simulink model "p3_rakete"  (R2015a)
settings: Solver=ode45  StartTime=0.0  StopTime=10.0  RelTol=1e-3
settings Model: Creator=leon  LastModifiedBy=leon

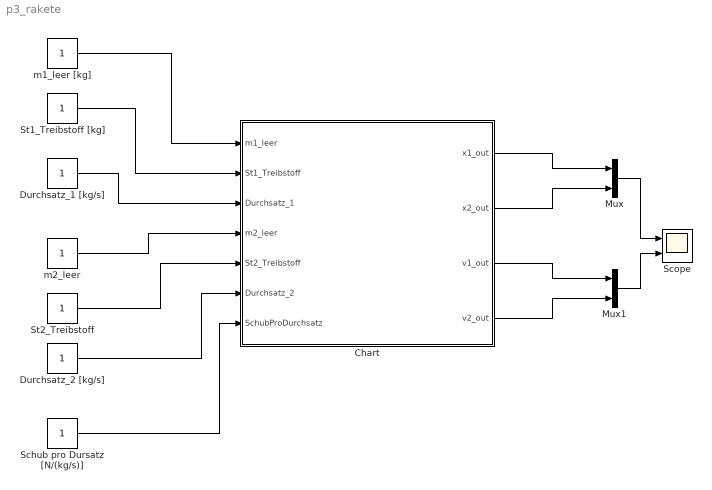
== system p3_rakete ==
  Chart : Stateflow chart  TreatAsAtomicUnit=on
  Durchsatz_1 [kg/s] : Constant
  Durchsatz_2 [kg/s] : Constant
  Mux : Mux  Inputs=2
  Mux1 : Mux  Inputs=2
  "Schub pro Dursatz [N/(kg/s)] " : Constant
  Scope : Scope  NumInputPorts=2
      settings: YMin=-5~-5  YMax=5~5
  St1_Treibstoff [kg] : Constant
  St2_Treibstoff : Constant
  "m1_leer [kg] " : Constant
  m2_leer : Constant
  wires:
  "m1_leer [kg] "/1 -> Chart/1(m1_leer)
  St1_Treibstoff [kg]/1 -> Chart/2(St1_Treibstoff)
  Durchsatz_1 [kg/s]/1 -> Chart/3(Durchsatz_1)
  m2_leer/1 -> Chart/4(m2_leer)
  St2_Treibstoff/1 -> Chart/5(St2_Treibstoff)
  Durchsatz_2 [kg/s]/1 -> Chart/6(Durchsatz_2)
  "Schub pro Dursatz [N/(kg/s)] "/1 -> Chart/7(SchubProDurchsatz)
  Chart/1(x1_out) -> Mux/1
  Chart/2(x2_out) -> Mux/2
  Chart/3(v1_out) -> Mux1/1
  Chart/4(v2_out) -> Mux1/2
  Mux/1 -> Scope/1
  Mux1/1 -> Scope/2

== stateflow chart p3_rakete/Chart ==
  settings: updateMethod=CONTINUOUS
  state StufenGemeinsam
    du:
    //Derivates
    [v1_dot; v2_dot] = Acc1();
    x1_dot = v1; x2_dot = v2;
    m1_dot = - Durchsatz1; m2_dot = 0;
    //Output
    x1_out = x1; x2_out = x2;
    v1_out = v1; v2_out = v2;
  state StufenGetrennt
  state Stufe2Ausgebrannt
  (default) -> StufenGemeinsam : {Init();}
  StufenGemeinsam -> StufenGetrennt
  StufenGetrennt -> Stufe2Ausgebrannt
  data: a1 function_output double; a2 function_output double; a1 function_output double; a2 function_output double; a1 function_output double; a2 function_output double; m1_leer input; St1_Treibstoff input; Durchsatz_1 input; m2_leer input; St2_Treibstoff input; Durchsatz_2 input; SchubProDurchsatz input; x1_out output; x2_out output; v1_out output; v2_out output; x1 local; v1 local; x2 local; v2 local; m1 local; m2 local; Erdmasse__kg_ constant double =5.9736*10^24; Erdradius__km_ constant double =6378; Gravitationskonstante constant double =66.743*10^12
  data x1 settings: updateMethod=SF_CONTINUOUS_TIME_DATA
  data v1 settings: updateMethod=SF_CONTINUOUS_TIME_DATA
  data x2 settings: updateMethod=SF_CONTINUOUS_TIME_DATA
  data v2 settings: updateMethod=SF_CONTINUOUS_TIME_DATA
  data m1 settings: updateMethod=SF_CONTINUOUS_TIME_DATA
  data m2 settings: updateMethod=SF_CONTINUOUS_TIME_DATA
  function Init:
    | function Init
    |  
    | %Leergewicht + Gewicht des Treibstoffes
    | m1 = m1_leer + St1_Treibstoff;
    | m2 = m2_leer + St2_Treibstoff;
    | 
    | %Die Rakete bewegt sich nicht.
    | v1 = 0;
    | v2 = 0;
  function [a1,a2] = Acc1:
    | function [a1,a2] = Acc1
  function [a1,a2] = Acc2:
    | function [a1,a2] = Acc2
  function [a1,a2] = Acc3:
    | function [a1,a2] = Acc3
